simulink subsystem "Cqdot_q_SubSystem"  (R2020b)
settings: Solver=VariableStepAuto  StartTime=0.0  StopTime=10.0  RelTol=1e-3
undefined symbols (not defined in the file or in its folder): l, mb, mrot, r, Ts, zbrot
settings Model: Creator=umberto  LastModifiedBy=umberto

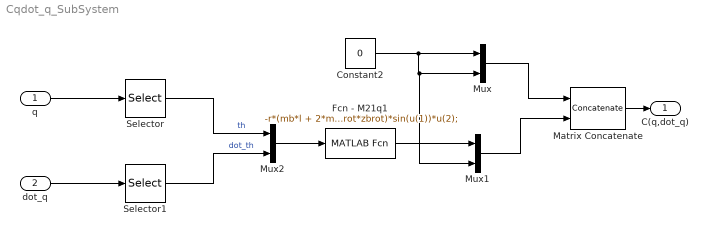
== system Cqdot_q_SubSystem ==
  q : Inport
  dot_q : Inport  Port=2
  Constant2 : Constant  Value=0  SampleTime=Ts
  Fcn - M21q1 : MATLABFcn  MATLABFcn=-r*(mb*l + 2*mrot*zbrot)*sin(u(1))*u(2);
  Matrix Concatenate : Concatenate  Mode=Multidimensional array  ConcatenateDimension=2
  Mux : Mux  Inputs=2
  Mux1 : Mux  Inputs=2
  Mux2 : Mux  Inputs=2
  Selector : Selector  InputPortWidth=2  IndexOptions=Index vector (dialog)  Indices=[2]  OutputSizes=1
  Selector1 : Selector  InputPortWidth=2  IndexOptions=Index vector (dialog)  Indices=[2]  OutputSizes=1
  C(q,dot_q) : Outport
  wires:
  Matrix Concatenate/1 -> C(q,dot_q)/1
  Mux1/1 -> Matrix Concatenate/2
  Mux/1 -> Matrix Concatenate/1
  Selector/1 -> Mux2/1  "th"
  q/1 -> Selector/1
  dot_q/1 -> Selector1/1
  Selector1/1 -> Mux2/2  "dot_th"
  Mux2/1 -> Fcn - M21q1/1
  Constant2/1 -> Mux1/2, Mux/2, Mux/1
  Fcn - M21q1/1 -> Mux1/1
